simulink model "SMC_Maglev"  (Simulink 9.2)
settings: Solver=ode1  StartTime=0.0  StopTime=1  FixedStep=0.0001  RelTol=1e-3
model workspace (MAT data in the model file):
  C = 0.00014
  g = 9.81
  m : num (value not decoded)
settings Model: Creator=piyus  LastModifiedBy=piyus
settings DataIOCC: LimitDataPoints=off  SaveFormat=Dataset  SignalLoggingSaveFormat=Dataset  ReturnWorkspaceOutputs=on
settings OptimizationCC: LifeSpan=auto
settings DebuggingCC: UnderspecifiedInitializationDetection=Simplified  MergeDetectMultiDrivingBlocksExec=error  FcnCallInpInsideContextMsg=error  StateNameClashWarn=none  SFUnexpectedBacktrackingDiag=error  SFNoUnconditionalDefaultTransitionDiag=error  SFExecutionAtInitializationDiag=warning  SFMachineParentedDataDiag=error
settings HardwareCC: ProdBitPerPointer=64  ProdBitPerSizeT=64  ProdBitPerPtrDiffT=64  ProdLargestAtomicFloat=Float  ProdIntDivRoundTo=Zero  ProdEndianess=LittleEndian  ProdWordSize=64  ProdHWDeviceType=Intel->x86-64 (Windows64)
settings ModelReferenceCC: PropagateSignalLabelsOutOfModel=on
settings SFSimCC: SimUseLocalCustomCode=on
settings RTWCC: RTWUseLocalCustomCode=on
settings CodeAppCC: StateflowObjectComments=off
settings GRTTargetCC: TargetLangStandard=C99 (ISO)  CombineOutputUpdateFcns=on  GRTInterface=off
settings ConfigComp: CovMetricSettings=dwe  CovSaveCumulativeToWorkspaceVar=off  CovSaveSingleToWorkspaceVar=off  CovExternalEMLEnable=on

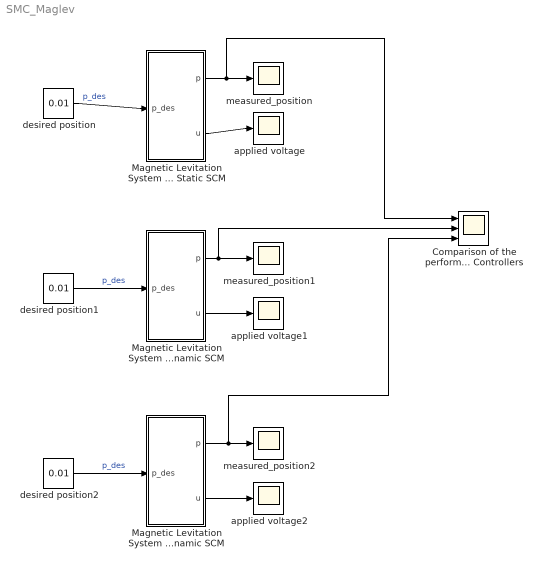
== system SMC_Maglev ==
  Comparison of the performance of the 3 Controllers : Scope  NumInputPorts=3
  Magnetic Levitation System with Dynamic SCM : Subsystem
  Magnetic Levitation System with Modified Dynamic SCM : Subsystem
  Magnetic Levitation System with Static SCM : Subsystem
  applied voltage : Scope
  applied voltage1 : Scope
  applied voltage2 : Scope
  desired position : Constant  Value=0.01
  desired position1 : Constant  Value=0.01
  desired position2 : Constant  Value=0.01
  measured_position : Scope
  measured_position1 : Scope
  measured_position2 : Scope
  wires:
  desired position/1 -> Magnetic Levitation System with Static SCM/1(p_des)  "p_des"
  Magnetic Levitation System with Static SCM/1(p) -> Comparison of the performance of the 3 Controllers/1, measured_position/1
  Magnetic Levitation System with Static SCM/2(u) -> applied voltage/1
  Magnetic Levitation System with Dynamic SCM/2(u) -> applied voltage1/1
  Magnetic Levitation System with Dynamic SCM/1(p) -> Comparison of the performance of the 3 Controllers/2, measured_position1/1
  desired position1/1 -> Magnetic Levitation System with Dynamic SCM/1(p_des)  "p_des"
  Magnetic Levitation System with Modified Dynamic SCM/2(u) -> applied voltage2/1
  Magnetic Levitation System with Modified Dynamic SCM/1(p) -> Comparison of the performance of the 3 Controllers/3, measured_position2/1
  desired position2/1 -> Magnetic Levitation System with Modified Dynamic SCM/1(p_des)  "p_des"

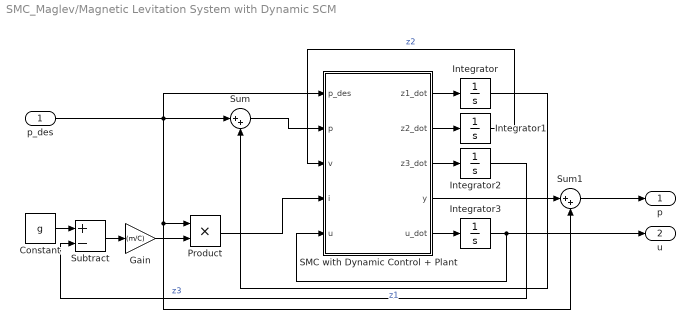
== system SMC_Maglev/Magnetic Levitation System with Dynamic SCM ==
  p_des : Inport
  Constant : Constant  Value=g
  Gain : Gain  Gain=(m/C)
  Integrator : Integrator  InitialCondition=0.008
  Integrator1 : Integrator
  Integrator2 : Integrator  InitialCondition=9
  Integrator3 : Integrator  InitialCondition=20
  Product : Product
  SMC with Dynamic Control + Plant : MATLAB Function  TreatAsAtomicUnit=on
  Subtract : Sum  Inputs=+-
  Sum : Sum  Inputs=|++
  Sum1 : Sum  Inputs=|++
  p : Outport
  u : Outport  Port=2
  wires:
  Product/1 -> SMC with Dynamic Control + Plant/4(i)
  Sum/1 -> SMC with Dynamic Control + Plant/2(p)
  p_des/1 -> Sum1/2, Product/1, SMC with Dynamic Control + Plant/1(p_des), Sum/1
  SMC with Dynamic Control + Plant/1(z1_dot) -> Integrator/1
  SMC with Dynamic Control + Plant/3(z3_dot) -> Integrator2/1
  Integrator2/1 -> Subtract/2  "z3"
  Gain/1 -> Product/2
  SMC with Dynamic Control + Plant/2(z2_dot) -> Integrator1/1
  Sum1/1 -> p/1
  Subtract/1 -> Gain/1
  Integrator1/1 -> SMC with Dynamic Control + Plant/3(v)  "z2"
  Constant/1 -> Subtract/1
  Integrator/1 -> Sum/2  "z1"
  SMC with Dynamic Control + Plant/4(y) -> Sum1/1
  SMC with Dynamic Control + Plant/5(u_dot) -> Integrator3/1
  Integrator3/1 -> SMC with Dynamic Control + Plant/5(u), u/1

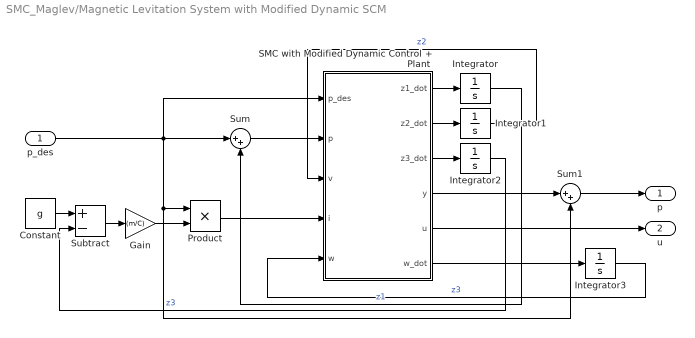
== system SMC_Maglev/Magnetic Levitation System with Modified Dynamic SCM ==
  p_des : Inport
  Constant : Constant  Value=g
  Gain : Gain  Gain=(m/C)
  Integrator : Integrator  InitialCondition=0.008
  Integrator1 : Integrator
  Integrator2 : Integrator  InitialCondition=9
  Integrator3 : Integrator
  Product : Product
  SMC with Modified Dynamic Control + Plant : MATLAB Function  TreatAsAtomicUnit=on
  Subtract : Sum  Inputs=+-
  Sum : Sum  Inputs=|++
  Sum1 : Sum  Inputs=|++
  p : Outport
  u : Outport  Port=2
  wires:
  Product/1 -> SMC with Modified Dynamic Control + Plant/4(i)
  Sum/1 -> SMC with Modified Dynamic Control + Plant/2(p)
  p_des/1 -> Sum1/2, Product/1, SMC with Modified Dynamic Control + Plant/1(p_des), Sum/1
  SMC with Modified Dynamic Control + Plant/1(z1_dot) -> Integrator/1
  SMC with Modified Dynamic Control + Plant/3(z3_dot) -> Integrator2/1
  Integrator2/1 -> Subtract/2  "z3"
  Gain/1 -> Product/2
  SMC with Modified Dynamic Control + Plant/2(z2_dot) -> Integrator1/1
  Sum1/1 -> p/1
  Subtract/1 -> Gain/1
  Integrator1/1 -> SMC with Modified Dynamic Control + Plant/3(v)  "z2"
  Constant/1 -> Subtract/1
  Integrator/1 -> Sum/2  "z1"
  SMC with Modified Dynamic Control + Plant/4(y) -> Sum1/1
  SMC with Modified Dynamic Control + Plant/5(u) -> u/1
  SMC with Modified Dynamic Control + Plant/6(w_dot) -> Integrator3/1
  Integrator3/1 -> SMC with Modified Dynamic Control + Plant/5(w)  "z3"

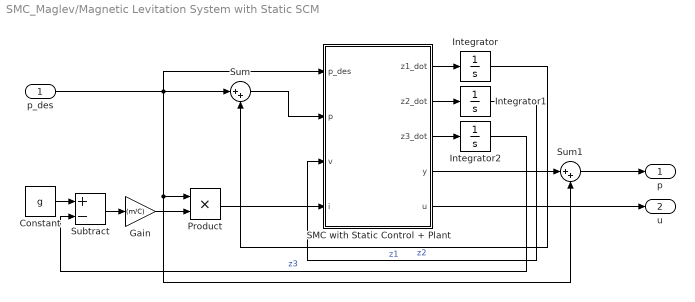
== system SMC_Maglev/Magnetic Levitation System with Static SCM ==
  p_des : Inport
  Constant : Constant  Value=g
  Gain : Gain  Gain=(m/C)
  Integrator : Integrator  InitialCondition=0.008
  Integrator1 : Integrator
  Integrator2 : Integrator  InitialCondition=9
  Product : Product
  SMC with Static Control + Plant : MATLAB Function  TreatAsAtomicUnit=on
  Subtract : Sum  Inputs=+-
  Sum : Sum  Inputs=|++
  Sum1 : Sum  Inputs=|++
  p : Outport
  u : Outport  Port=2
  wires:
  Product/1 -> SMC with Static Control + Plant/4(i)
  Sum/1 -> SMC with Static Control + Plant/2(p)
  p_des/1 -> Sum1/2, Product/1, SMC with Static Control + Plant/1(p_des), Sum/1
  SMC with Static Control + Plant/1(z1_dot) -> Integrator/1
  SMC with Static Control + Plant/3(z3_dot) -> Integrator2/1
  Integrator2/1 -> Subtract/2  "z3"
  Gain/1 -> Product/2
  SMC with Static Control + Plant/2(z2_dot) -> Integrator1/1
  Sum1/1 -> p/1
  Subtract/1 -> Gain/1
  Integrator1/1 -> SMC with Static Control + Plant/3(v)  "z2"
  Constant/1 -> Subtract/1
  Integrator/1 -> Sum/2  "z1"
  SMC with Static Control + Plant/4(y) -> Sum1/1
  SMC with Static Control + Plant/5(u) -> u/1

== matlab function Magnetic Levitation System with Dynamic SCM/SMC with Dynamic Control + Plant ==
  data: p_des input double; z1_dot output double; z2_dot output double; z3_dot output double; p input double; y output double; v input double; i input double; u_dot output double; u input double
function [z1_dot, z2_dot, z3_dot, y, u_dot]= fcn(p_des, p, v, i, u)

%%
% x1 = p (position)
% x2 = v (velocity)
% x3 = i (current)
% u = e (applied voltage)

g = 9.81;
C = 1.4*10^-4; 
R = 28.7;
L1 = 0.65;
m = 11.87*10^-3;

tau = 50000;
m1 = 93;
m2 = 2882;
m3 = 29760;

L = L1 + 2*C/p;

% Defining State variables
x1 = p;
x2 = v;
x3 = i;
x1_des = p_des;

z1 = x1 - x1_des;
z2 = x2;                   % x2_des = 0
z3 = g - (C/m)*(x3/x1)^2;   

f1 = 2*(C/m)*((1 - 2*C/(L*x1))*x2*x3^2/x1^3 + (R/L)*(x3^2/x1^2));
g1 = -2*C*x3/(L*m*x1^2);

f1_dot = 2*(C/m)*(-2*R^2*x3^2/(L^2*x1^2) + (g - 4*R*x2/L)*(x3^2/x1^3) + (10*R*C*x2/L^2 - 3*x2^2 - 2*C*g/L)*(x3^2/x1^4) + (12*C*x2^2/L - C*x3^2/m)*(x3^2/x1^5) + (2*C^2*x3^2/(L*m) - 12*C^2*x2^2/L^2)*(x3^2/x1^6) + (2*x2/(L*x1) - 4*C*x2/(L^2*x1^2) + 2*R/L^2)*x3*u/x1^2);
g1_dot = (-R/L -2*x2/x1 + 4*C*x2/(L*x1^2))*g1 - 2*C*u/(m*L^2*x1^2);

u_dot = 1/g1*(-f1_dot - g1_dot*u - m1*(f1 + g1*u) - m2*z3 - m3*z2 - tau*sign(f1 + g1*u + m1*z3 + m2*z2 + m3*z1)); % Control input : applied voltage

% State space model in new coordinates. 
z1_dot = z2;
z2_dot = z3;
z3_dot = f1 + g1*u;

y = z1; % Output of state space model.

== matlab function Magnetic Levitation System with Static SCM/SMC with Static Control + Plant ==
  data: p_des input double; z1_dot output double; z2_dot output double; z3_dot output double; p input double; y output double; v input double; i input double; u output double
function [z1_dot, z2_dot, z3_dot, y, u]= fcn(p_des, p, v, i)

%%
% x1 = p (position)
% x2 = v (velocity)
% x3 = i (current)
% u = e (applied voltage)

g = 9.81;
C = 1.4*10^-4; 
R = 28.7;
L1 = 0.65;
m = 11.87*10^-3  ;

W = 350;
lambda_1 = 61;
lambda_2 = 930;

L = L1 + 2*C/p;

% Defining State variables
x1 = p;
x2 = v;
x3 = i;
x1_des = p_des;

z1 = x1 - x1_des;
z2 = x2;                   % x2_des = 0
z3 = g - (C/m)*(x3/x1)^2;   

f1 = 2*(C/m)*((1 - 2*C/(L*x1))*x2*x3^2/x1^3 + (R/L)*(x3^2/x1^2));
g1 = -2*C*x3/(L*m*x1^2);

u = 1/g1*(-f1 - lambda_1*z3 - lambda_2*z2 - W*sign(z3 + lambda_1*z2 + lambda_2*z1)); % Control input : applied voltage

% State space model in new coordinates. 
z1_dot = z2;
z2_dot = z3;
z3_dot = f1 + g1*u;

y = z1; % Output of state space model.

== matlab function Magnetic Levitation System with Modified Dynamic SCM/SMC with Modified Dynamic Control + Plant ==
  data: p_des input double; z1_dot output double; z2_dot output double; z3_dot output double; p input double; y output double; v input double; i input double; u output double; w input double; w_dot output double
function [z1_dot, z2_dot, z3_dot, y, u, w_dot]= fcn(p_des, p, v, i, w)

%%
% x1 = p (position)
% x2 = v (velocity)
% x3 = i (current)
% u = e (applied voltage)

g = 9.81;
C = 1.4*10^-4; 
R = 28.7;
L1 = 0.65;
m = 11.87*10^-3;

W2 = 100;
c1 = 29760;
c2 = 2882;
c3 = 93;

L = L1 + 2*C/p;

% Defining State variables
x1 = p;
x2 = v;
x3 = i;
x1_des = p_des;

z1 = x1 - x1_des;
z2 = x2;                   % x2_des = 0
z3 = g - (C/m)*(x3/x1)^2;   

f1 = 2*(C/m)*((1 - 2*C/(L*x1))*x2*x3^2/x1^3 + (R/L)*(x3^2/x1^2));
g1 = -2*C*x3/(L*m*x1^2);

u = -1/g1*(f1 + c1*z1 + c2*z2 + c3*z3) + w; % Control input : applied voltage
w_dot = -W2*sign(u + 1/g1*(f1 + c1*z1 + c2*z2 + c3*z3));

% State space model in new coordinates. 
z1_dot = z2;
z2_dot = z3;
z3_dot = f1 + g1*u;

y = z1; % Output of state space model.
